simulink model "reactormdlv1"  (R2020a)
settings: Solver=VariableStepAuto  StartTime=0.0  StopTime=2.4  RelTol=1e-3
settings Model: Creator=marce  LastModifiedBy=marce

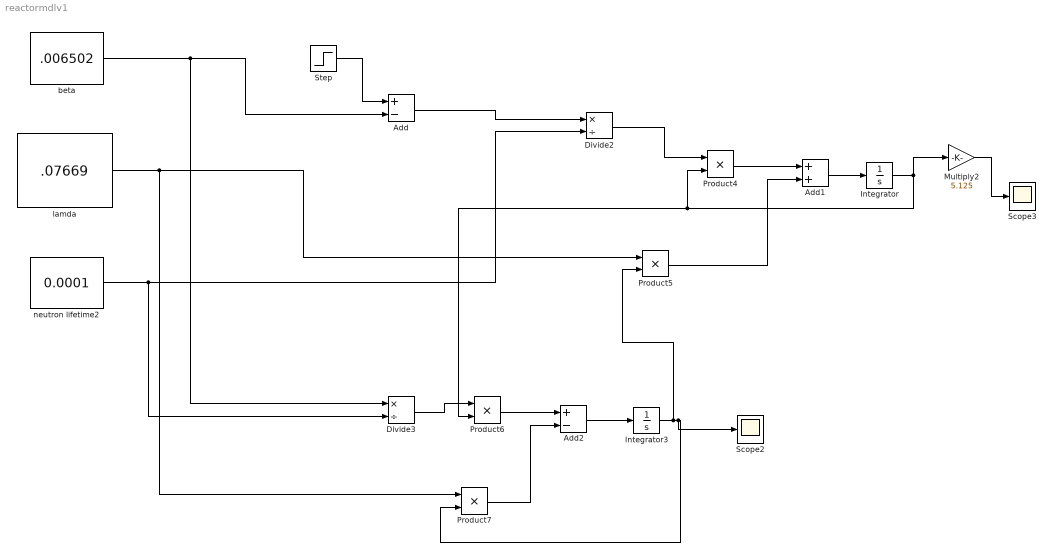
== system reactormdlv1 ==
  Add : Sum  Inputs=+-
  Add1 : Sum
  Add2 : Sum  Inputs=+-
  Divide2 : Product  Inputs=*/
  Divide3 : Product  Inputs=*/
  Integrator : Integrator
  Integrator3 : Integrator  InitialCondition=1695.658
  Multiply2 : Gain  Gain=5.125
  Product{4..7} (4 alike) : Product
  Scope2 : Scope
  Scope3 : Scope
  Step : Step  After=.006502*.3  SampleTime=0
  beta : Constant  Value=.006502
  lamda : Constant  Value=.07669
  neutron lifetime2 : Constant  Value=0.0001
  wires:
  beta/1 -> Divide3/1, Add/2
  Add/1 -> Divide2/1
  neutron lifetime2/1 -> Divide3/2, Divide2/2
  Divide2/1 -> Product4/1
  Product4/1 -> Add1/1
  lamda/1 -> Product7/1, Product5/1
  Product5/1 -> Add1/2
  Add1/1 -> Integrator/1
  Integrator/1 -> Product6/2, Product4/2, Multiply2/1
  Divide3/1 -> Product6/1
  Product6/1 -> Add2/1
  Product7/1 -> Add2/2
  Add2/1 -> Integrator3/1
  Integrator3/1 -> Product5/2, Scope2/1, Product7/2
  Step/1 -> Add/1
  Multiply2/1 -> Scope3/1
